simulink model "model_base_bros"  (R2017b)
settings: Solver=FixedStepDiscrete  StartTime=0.0  StopTime=inf  FixedStep=sampleTime  RelTol=1e-3
PostLoadFcn:
  | % load model parameters
  | % pname = fileparts(get_param('model_base_bros','filename'));
  | % run([pname  '\parameters_base_model_bros.m']);
  | parameters_base_model_bros;
  | 
  | % set requested state
  | set_param('model_base_bros/Requested state','Value',num2str(0));
InitFcn:
  | % load model parameters
  | % pname = fileparts(get_param('model_base_bros','filename'));
  | % run([pname  '\parameters_base_model_bros.m']);
  | parameters_base_model_bros;
  | 
  | % set requested state
  | set_param('model_base_bros/Requested state','Value',num2str(0));
StartFcn:
  | % load model parameters
  | % pname = fileparts(get_param('model_base_bros','filename'));
  | % run([pname  '\parameters_base_model_bros.m']);
  | parameters_base_model_bros;
  | 
  | % set requested state
  | set_param('model_base_bros/Requested state','Value',num2str(0));
StopFcn:
  | % switch off data logger (to hopefully avoid corrupt files). TwinCAT doesn't properly switch off the logger when shutting down the model
  | % no idea if this'll work.
  | set_param('model_base_bros/Record data (1 = yes, 0 = no)','Value',num2str(0));
values from neighbouring files (symbols this model uses):
  FFMatrix = -[0 -15; 15 0]    [parameters_base_model_bros.m]
  Lb = 0.07    [parameters_base_model_bros.m]
  Lf = 0.238    [parameters_base_model_bros.m]
  Lu = 0.153    [parameters_base_model_bros.m]
  sampleTime = 0.001    [parameters_base_model_bros.m]
undefined symbols (not defined in the file or in its folder): BROS1, BROS2
libraries: simulink x27, LibraryFM x14, VariousBlocksLibrary x7, simulink_extras x1
(part 1 of 3)
settings Model: SimulationMode=external  Creator=niekbeckers  LastModifiedBy=TCUser
settings DataIOCC: LimitDataPoints=on  SaveFormat=Array
settings OptimizationCC: BlockReduction=off  BooleanDataType=off  LocalBlockOutputs=off  LifeSpan=inf
settings DebuggingCC: SaveWithParameterizedLinksMsg=none  UnderspecifiedInitializationDetection=Classic  MergeDetectMultiDrivingBlocksExec=none  SignalResolutionControl=TryResolveAllWithWarning  SFUnexpectedBacktrackingDiag=warning  SFNoUnconditionalDefaultTransitionDiag=warning  SFExecutionAtInitializationDiag=none
settings HardwareCC: ProdBitPerPointer=32  ProdBitPerSizeT=32  ProdBitPerPtrDiffT=32  ProdLargestAtomicFloat=None  ProdIntDivRoundTo=Undefined  ProdEndianess=Unspecified  ProdWordSize=32  ProdHWDeviceType=32-bit Generic  TargetBitPerPointer=64  TargetBitPerSizeT=64  TargetBitPerPtrDiffT=64  TargetLongLongMode=on  TargetIntDivRoundTo=Zero  TargetEndianess=LittleEndian  TargetWordSize=64  TargetHWDeviceType=MATLAB Host  ProdEqTarget=off
settings ModelReferenceCC: PropagateSignalLabelsOutOfModel=off
settings RTWCC: SystemTargetFile=TwinCAT.tlc  GenCodeOnly=on  MakeCommand=make_tct  TemplateMakefile=tct_msbuild.tmf  Description=TwinCAT Target  GenerateReport=on  TargetLang=C++
settings CodeAppCC: StateflowObjectComments=on
settings STFCustomTargetCC: CompOptLevelCompliant=on  GeneratePreprocessorConditionals=Disable all  MATLABClassNameForMDSCustomization=Simulink.SoftwareTarget.TargetSpecificTriggerConfigurationBase  SystemTargetFile=TwinCAT.tlc
settings ConfigComp: CovMetricSettings=dw  CovHtmlReporting=on  CovSaveCumulativeToWorkspaceVar=on  CovSaveSingleToWorkspaceVar=on  CovExternalEMLEnable=off  CovSFcnEnable=off
settings SimscapeCC: SimscapeNormalizeSystem=off

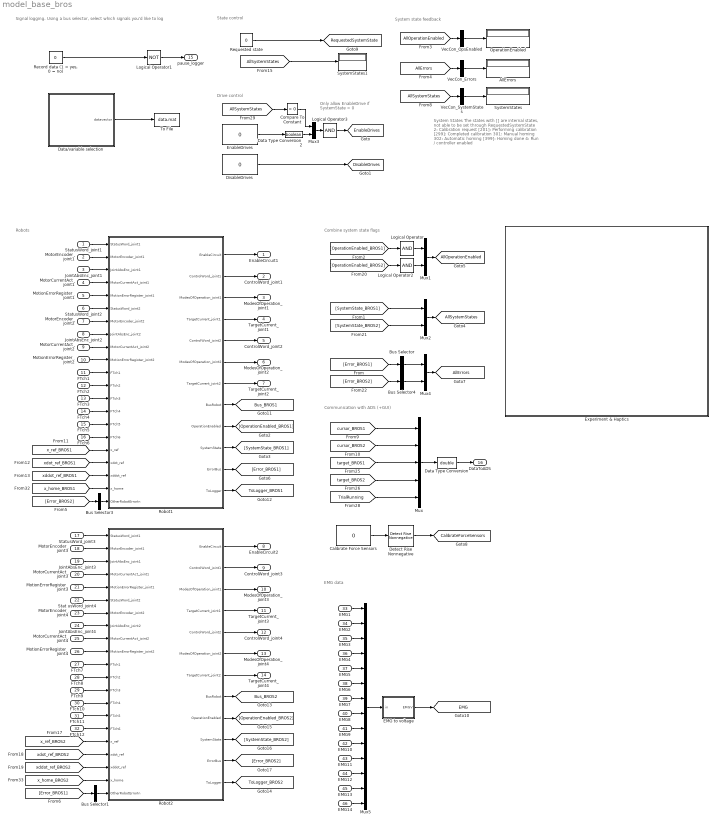
== system model_base_bros ==
  note: EMG data
  note: Drive control
  note: System state feedback
  note: Only allow EnableDrive
      | if SystemState > 0
  note: Communication with ADS (+GUI)
  note: Signal logging.
      | Using a bus selector, select which signals you'd like to log
  note: System States
      | The states with [] are internal states, not able to be set through RequestedSystemState
      | 2: Calibration request
      | [201]: Performing calibration
      | [299]: Completed calibration
      | 301: Manual homing
      | 302: Automatic homing
      | [399]: Homing done
      | 4: Run / controller enabled
  note: State control
  note: Combine system state flags
  note: Robots
  StatusWord_joint1 : Inport  OutDataTypeStr=uint16  PortDimensions=1
  MotorEncoder_joint1 : Inport  Port=2  OutDataTypeStr=int32  PortDimensions=1
  JointAbsEnc_joint1 : Inport  Port=3  OutDataTypeStr=int32  PortDimensions=1
  MotorCurrentAct_joint1 : Inport  Port=4  OutDataTypeStr=int16  PortDimensions=1
  MotionErrorRegister_joint1 : Inport  Port=5  OutDataTypeStr=uint16  PortDimensions=1
  StatusWord_joint2 : Inport  Port=6  OutDataTypeStr=uint16  PortDimensions=1
  MotorEncoder_joint2 : Inport  Port=7  OutDataTypeStr=int32  PortDimensions=1
  JointAbsEnc_joint2 : Inport  Port=8  OutDataTypeStr=int32  PortDimensions=1
  MotorCurrentAct_joint2 : Inport  Port=9  OutDataTypeStr=int16  PortDimensions=1
  MotionErrorRegister_joint2 : Inport  Port=10  OutDataTypeStr=uint16  PortDimensions=1
  FTch1 : Inport  Port=11  OutDataTypeStr=single  PortDimensions=1
  FTch2 : Inport  Port=12  OutDataTypeStr=single  PortDimensions=1
  FTch3 : Inport  Port=13  OutDataTypeStr=single  PortDimensions=1
  FTch4 : Inport  Port=14  OutDataTypeStr=single  PortDimensions=1
  FTch5 : Inport  Port=15  OutDataTypeStr=single  PortDimensions=1
  FTch6 : Inport  Port=16  OutDataTypeStr=single  PortDimensions=1
  StatusWord_joint3 : Inport  Port=17  OutDataTypeStr=uint16  PortDimensions=1
  MotorEncoder_joint3 : Inport  Port=18  OutDataTypeStr=int32  PortDimensions=1
  JointAbsEnc_joint3 : Inport  Port=19  OutDataTypeStr=int32  PortDimensions=1
  MotorCurrentAct_joint3 : Inport  Port=20  OutDataTypeStr=int16  PortDimensions=1
  MotionErrorRegister_joint3 : Inport  Port=21  OutDataTypeStr=uint16  PortDimensions=1
  Stat usWord_joint4 : Inport  Port=22  OutDataTypeStr=uint16  PortDimensions=1
  MotorEncoder_joint4 : Inport  Port=23  OutDataTypeStr=int32  PortDimensions=1
  JointAbsEnc_joint4 : Inport  Port=24  OutDataTypeStr=int32  PortDimensions=1
  MotorCurrentAct_joint4 : Inport  Port=25  OutDataTypeStr=int16  PortDimensions=1
  MotionErrorRegister_joint4 : Inport  Port=26  OutDataTypeStr=uint16  PortDimensions=1
  FTch7 : Inport  Port=27  OutDataTypeStr=single  PortDimensions=1
  FTch8 : Inport  Port=28  OutDataTypeStr=single  PortDimensions=1
  FTch9 : Inport  Port=29  OutDataTypeStr=single  PortDimensions=1
  FTch10 : Inport  Port=30  OutDataTypeStr=single  PortDimensions=1
  FTch11 : Inport  Port=31  OutDataTypeStr=single  PortDimensions=1
  FTch12 : Inport  Port=32  OutDataTypeStr=single  PortDimensions=1
  EMG1 : Inport  Port=33  OutDataTypeStr=int16  PortDimensions=1
  EMG2 : Inport  Port=34  OutDataTypeStr=int16  PortDimensions=1
  EMG3 : Inport  Port=35  OutDataTypeStr=int16  PortDimensions=1
  EMG4 : Inport  Port=36  OutDataTypeStr=int16  PortDimensions=1
  EMG5 : Inport  Port=37  OutDataTypeStr=int16  PortDimensions=1
  EMG6 : Inport  Port=38  OutDataTypeStr=int16  PortDimensions=1
  EMG7 : Inport  Port=39  OutDataTypeStr=int16  PortDimensions=1
  EMG8 : Inport  Port=40  OutDataTypeStr=int16  PortDimensions=1
  EMG9 : Inport  Port=41  OutDataTypeStr=int16  PortDimensions=1
  EMG10 : Inport  Port=42  OutDataTypeStr=int16  PortDimensions=1
  EMG11 : Inport  Port=43  OutDataTypeStr=int16  PortDimensions=1
  EMG12 : Inport  Port=44  OutDataTypeStr=int16  PortDimensions=1
  EMG13 : Inport  Port=45  OutDataTypeStr=int16  PortDimensions=1
  EMG14 : Inport  Port=46  OutDataTypeStr=int16  PortDimensions=1
  AllErrors : Display
      settings: OpenFcn=msgbox(DecodeBROSError(gcb));  Format=hex (Stored Integer)
  Bus Selector : BusSelector  OutputSignals=ErrorCodeLatched  OutputAsBus=on
  Bus Selector1 : BusSelector  OutputSignals=ErrorCode  OutputAsBus=on
  Bus Selector3 : BusSelector  OutputSignals=ErrorCode  OutputAsBus=on
  Bus Selector4 : BusSelector  OutputSignals=ErrorCodeLatched  OutputAsBus=on
  Calibrate Force Sensors : Constant  Value=0
      settings: OpenFcn=set_param(gcb,'Value','1');tname = ['toggletimer_' gcb];delete(timerfind('name',tname));t = timer('timerfcn', ['set_param(''',gcb,''',''Value'',''0'')'],'executionmode','singleshot','startdelay',1,'name',tname);start(t);
      mask Display: fprintf('PushToTrigger\n%s',get_param(gcb,'value'))
  Compare To Constant : simulink/Logic and Bit Operations/Compare To Constant  relop=>  const=0  OutDataTypeStr=boolean
  Data Type Conversion : DataTypeConversion  OutDataTypeStr=double
  Data Type Conversion2 : DataTypeConversion  OutDataTypeStr=boolean
  Data/variable selection : Subsystem
  Detect Rise Nonnegative : simulink/Logic and Bit Operations/Detect Rise Nonnegative  vinit=0  OutDataTypeStr=boolean
      settings: SourceProductName=Simulink  SourceProductBaseCode=SL
  DisableDrives : Constant  Value=0
      settings: OpenFcn=set_param(gcb,'Value','1');tname = ['toggletimer_' gcb];delete(timerfind('name',tname));t = timer('timerfcn', ['set_param(''',gcb,''',''Value'',''0'')'],'executionmode','singleshot','startdelay',1,'name',tname);start(t);
      mask Display: fprintf('PushToTrigger\n%s',get_param(gcb,'value'))
  EMG to voltage : MATLAB Function  TreatAsAtomicUnit=on
  EnableDrives : Constant  Value=0
      settings: OpenFcn=set_param(gcb,'Value','1');tname = ['toggletimer_' gcb];delete(timerfind('name',tname));t = timer('timerfcn', ['set_param(''',gcb,''',''Value'',''0'')'],'executionmode','singleshot','startdelay',1,'name',tname);start(t);
      mask Display: fprintf('PushToTrigger\n%s',get_param(gcb,'value'))
  Experiment & Haptics : Subsystem
  Logical Operator : Logic  Inputs=1  AllPortsSameDT=off  OutDataTypeStr=boolean
  Logical Operator1 : Logic  Operator=NOT  Inputs=1  AllPortsSameDT=off  OutDataTypeStr=boolean
  Logical Operator2 : Logic  Inputs=1  AllPortsSameDT=off  OutDataTypeStr=boolean
  Logical Operator3 : Logic  Inputs=1  AllPortsSameDT=off  OutDataTypeStr=boolean
  Mux : Mux  Inputs=5
  Mux{1..4} (4 alike) : Mux  Inputs=2
  Mux5 : Mux  Inputs=14
  OperationEnabled : Display
  "Record data (1 = yes, 0 = no)" : Constant  Value=0  OutDataTypeStr=boolean
  Requested state : Constant  Value=0
  Robot1 : Subsystem  mask{RobotStruct=BROS1}
      mask prompts: RobotStruct "Robot struct (data)"
  Robot2 : Subsystem  mask{RobotStruct=BROS2}
      mask prompts: RobotStruct "Robot struct (data)"
  SystemStates : Display
  SystemStates1 : Display
  To File : ToFile  Filename=data.mat  MatrixName=data
  VecCon_Errors : Concatenate  NumInputs=1
  VecCon_OpsEnabled : Concatenate  NumInputs=1
  VecCon_SystemStates : Concatenate  NumInputs=1
  EnableCircuit1 : Outport  OutDataTypeStr=boolean  PortDimensions=1
  ControlWord_joint1 : Outport  Port=2  OutDataTypeStr=uint16  PortDimensions=1
  ModesOfOperation_joint1 : Outport  Port=3  OutDataTypeStr=int8  PortDimensions=1
  TargetCurrent_joint1 : Outport  Port=4  OutDataTypeStr=int16  PortDimensions=1
  ControlWord_joint2 : Outport  Port=5  OutDataTypeStr=uint16  PortDimensions=1
  ModesOfOperation_joint2 : Outport  Port=6  OutDataTypeStr=int8  PortDimensions=1
  TargetCurrent_joint2 : Outport  Port=7  OutDataTypeStr=int16  PortDimensions=1
  EnableCircuit2 : Outport  Port=8  OutDataTypeStr=boolean  PortDimensions=1
  ControlWord_joint3 : Outport  Port=9  OutDataTypeStr=uint16  PortDimensions=1
  ModesOfOperation_joint3 : Outport  Port=10  OutDataTypeStr=int8  PortDimensions=1
  TargetCurrent_joint3 : Outport  Port=11  OutDataTypeStr=int16  PortDimensions=1
  ControlWord_joint4 : Outport  Port=12  OutDataTypeStr=uint16  PortDimensions=1
  ModesOfOperation_joint4 : Outport  Port=13  OutDataTypeStr=int8  PortDimensions=1
  TargetCurrent_joint4 : Outport  Port=14  OutDataTypeStr=int16  PortDimensions=1
  pause_logger : Outport  Port=15  OutDataTypeStr=boolean  PortDimensions=1
  DataToADS : Outport  Port=16  OutDataTypeStr=double
  tag scope: AllErrors=global, AllOperationEnabled=global, AllSystemStates=global, Bus_BROS1=global, Bus_BROS2=global, CalibrateForceSensors=global, DisableDrives=global, EMG=global, EnableDrives=global, RequestedSystemState=global, ToLogger_BROS1=global, ToLogger_BROS2=global
  wires:
  DisableDrives/1 -> [DisableDrives]
  Robot1/9(OperationEnabled) -> [OperationEnabled_BROS1]
  [AllOperationEnabled] -> VecCon_OpsEnabled/1
  Robot1/10(SystemState) -> [SystemState_BROS1]
  [SystemState_BROS1] -> Mux2/1
  Mux2/1 -> [AllSystemStates]
  Mux1/1 -> [AllOperationEnabled]
  [OperationEnabled_BROS1] -> Logical Operator/1
  Robot1/11(ErrorBus) -> [Error_BROS1]
  [Error_BROS1] -> Bus Selector/1
  [AllErrors] -> VecCon_Errors/1
  [x_ref_BROS1] -> Robot1/17(x_ref)
  [xdot_ref_BROS1] -> Robot1/18(xdot_ref)
  [xddot_ref_BROS1] -> Robot1/19(xddot_ref)
  Requested state/1 -> [RequestedSystemState]
  Robot1/8(BusRobot) -> [Bus_BROS1]
  StatusWord_joint1/1 -> Robot1/1(StatusWord_joint1)
  MotorEncoder_joint1/1 -> Robot1/2(MotorEncoder_joint1)
  JointAbsEnc_joint1/1 -> Robot1/3(JointAbsEnc_joint1)
  MotorCurrentAct_joint1/1 -> Robot1/4(MotorCurrentAct_joint1)
  StatusWord_joint2/1 -> Robot1/6(StatusWord_joint2)
  MotorEncoder_joint2/1 -> Robot1/7(MotorEncoder_joint2)
  JointAbsEnc_joint2/1 -> Robot1/8(JointAbsEnc_joint2)
  MotorCurrentAct_joint2/1 -> Robot1/9(MotorCurrentAct_joint2)
  FTch1/1 -> Robot1/11(FTch1)
  FTch2/1 -> Robot1/12(FTch2)
  FTch3/1 -> Robot1/13(FTch3)
  FTch4/1 -> Robot1/14(FTch4)
  FTch5/1 -> Robot1/15(FTch5)
  FTch6/1 -> Robot1/16(FTch6)
  Robot1/2(ControlWord_joint1) -> ControlWord_joint1/1
  Robot1/3(ModesOfOperation_joint1) -> ModesOfOperation_joint1/1
  Robot1/4(TargetCurrent_joint1) -> TargetCurrent_joint1/1
  Robot1/7(TargetCurrent_joint2) -> TargetCurrent_joint2/1
  Robot1/6(ModesOfOperation_joint2) -> ModesOfOperation_joint2/1
  Robot1/5(ControlWord_joint2) -> ControlWord_joint2/1
  Robot1/12(ToLogger) -> [ToLogger_BROS1]
  Logical Operator/1 -> Mux1/1
  [AllSystemStates] -> SystemStates1/1
  Logical Operator1/1 -> pause_logger/1
  Robot2/9(OperationEnabled) -> [OperationEnabled_BROS2]
  Robot2/10(SystemState) -> [SystemState_BROS2]
  Robot2/11(ErrorBus) -> [Error_BROS2]
  [x_ref_BROS2] -> Robot2/17(x_ref)
  [xdot_ref_BROS2] -> Robot2/18(xdot_ref)
  [xddot_ref_BROS2] -> Robot2/19(xddot_ref)
  Robot2/8(BusRobot) -> [Bus_BROS2]
  StatusWord_joint3/1 -> Robot2/1(StatusWord_joint1)
  MotorEncoder_joint3/1 -> Robot2/2(MotorEncoder_joint1)
  JointAbsEnc_joint3/1 -> Robot2/3(JointAbsEnc_joint1)
  MotorCurrentAct_joint3/1 -> Robot2/4(MotorCurrentAct_joint1)
  Stat usWord_joint4/1 -> Robot2/6(StatusWord_joint2)
  MotorEncoder_joint4/1 -> Robot2/7(MotorEncoder_joint2)
  MotorCurrentAct_joint4/1 -> Robot2/9(MotorCurrentAct_joint2)
  FTch7/1 -> Robot2/11(FTch1)
  FTch8/1 -> Robot2/12(FTch2)
  FTch9/1 -> Robot2/13(FTch3)
  FTch10/1 -> Robot2/14(FTch4)
  FTch12/1 -> Robot2/16(FTch6)
  Robot2/1(EnableCircuit) -> EnableCircuit2/1
  Robot2/2(ControlWord_joint1) -> ControlWord_joint3/1
  Robot2/3(ModesOfOperation_joint1) -> ModesOfOperation_joint3/1
  Robot2/7(TargetCurrent_joint2) -> TargetCurrent_joint4/1
  Robot2/6(ModesOfOperation_joint2) -> ModesOfOperation_joint4/1
  Robot2/5(ControlWord_joint2) -> ControlWord_joint4/1
  Robot2/12(ToLogger) -> [ToLogger_BROS2]
  [OperationEnabled_BROS2] -> Logical Operator2/1
  Logical Operator2/1 -> Mux1/2
  [SystemState_BROS2] -> Mux2/2
  Mux4/1 -> [AllErrors]
  Bus Selector/1 -> Mux4/1
  [Error_BROS2] -> Bus Selector4/1
  Bus Selector4/1 -> Mux4/2
  Robot1/1(EnableCircuit) -> EnableCircuit1/1
  Robot2/4(TargetCurrent_joint1) -> TargetCurrent_joint3/1
  JointAbsEnc_joint4/1 -> Robot2/8(JointAbsEnc_joint2)
  FTch11/1 -> Robot2/15(FTch5)
  [Error_BROS2] -> Bus Selector3/1
  [Error_BROS1] -> Bus Selector1/1
  Bus Selector1/1 -> Robot2/21(OtherRobotErrorIn)
  Bus Selector3/1 -> Robot1/21(OtherRobotErrorIn)
  VecCon_Errors/1 -> AllErrors/1
  [AllSystemStates] -> VecCon_SystemStates/1
  VecCon_SystemStates/1 -> SystemStates/1
  VecCon_OpsEnabled/1 -> OperationEnabled/1
  Mux/1 -> Data Type Conversion/1
  Data Type Conversion/1 -> DataToADS/1
  [cursor_BROS1] -> Mux/1
  [cursor_BROS2] -> Mux/2
  [target_BROS1] -> Mux/3
  [target_BROS2] -> Mux/4
  [TrialRunning] -> Mux/5
  Calibrate Force Sensors/1 -> Detect Rise Nonnegative/1
  Detect Rise Nonnegative/1 -> [CalibrateForceSensors]
  [AllSystemStates] -> Compare To Constant/1
  Logical Operator3/1 -> [EnableDrives]
  EnableDrives/1 -> Data Type Conversion2/1
  Compare To Constant/1 -> Mux3/1
  Mux3/1 -> Logical Operator3/1
  Data Type Conversion2/1 -> Mux3/2
  [x_home_BROS1] -> Robot1/20(x_home)
  [x_home_BROS2] -> Robot2/20(x_home)
  Data/variable selection/1(datavector) -> To File/1
  MotionErrorRegister_joint1/1 -> Robot1/5(MotionErrorRegister_joint1)
  MotionErrorRegister_joint2/1 -> Robot1/10(MotionErrorRegister_joint2)
  MotionErrorRegister_joint3/1 -> Robot2/5(MotionErrorRegister_joint1)
  MotionErrorRegister_joint4/1 -> Robot2/10(MotionErrorRegister_joint2)
  EMG1/1 -> Mux5/1
  EMG2/1 -> Mux5/2
  EMG3/1 -> Mux5/3
  EMG4/1 -> Mux5/4
  EMG5/1 -> Mux5/5
  EMG6/1 -> Mux5/6
  EMG7/1 -> Mux5/7
  EMG8/1 -> Mux5/8
  EMG9/1 -> Mux5/9
  EMG10/1 -> Mux5/10
  EMG11/1 -> Mux5/11
  EMG12/1 -> Mux5/12
  Mux5/1 -> EMG to voltage/1(in)
  EMG to voltage/1(EMGV) -> [EMG]
  EMG13/1 -> Mux5/13
  EMG14/1 -> Mux5/14
  "Record data (1 = yes, 0 = no)"/1 -> Logical Operator1/1

== system model_base_bros/Data//variable selection ==
  Bus to Vector : BusToVector
  Bus to Vector3 : BusToVector
  BusSelectorLoggerBROS1 : BusSelector  OutputSignals=SystemState,qJointSpace.q_AbsEnc,qJointSpace.qdot_AbsEnc,qJointSpace.q_IncEnc,qJointSpace.qdot_IncEnc,xOpSpace.x_AbsEnc,xOpSpace.xdot_AbsEnc,xOpSpace.x,xOpSpace.xdot,Controller_ToLogger.x_ref,Controller_ToLogger.xdot_ref,Controller_ToLogger.xddot_ref,qJointSpace.JointTorque_Nm,BusFTSensor.ForcesOpSpace  OutputAsBus=on
  BusSelectorLoggerBROS2 : BusSelector  OutputSignals=SystemState,qJointSpace.q_AbsEnc,qJointSpace.qdot_AbsEnc,qJointSpace.q_IncEnc,qJointSpace.qdot_IncEnc,xOpSpace.x_AbsEnc,xOpSpace.xdot_AbsEnc,xOpSpace.x,xOpSpace.xdot,Controller_ToLogger.x_ref,Controller_ToLogger.xdot_ref,Controller_ToLogger.xddot_ref,qJointSpace.JointTorque_Nm,BusFTSensor.ForcesOpSpace  OutputAsBus=on
  Constant : Constant  Value=0
  Mux : Mux  Inputs=6
  Mux5 : Mux  Inputs=13
  datavector : Outport
  wires:
  BusSelectorLoggerBROS1/1 -> Bus to Vector/1
  [ToLogger_BROS1] -> BusSelectorLoggerBROS1/1
  Bus to Vector3/1 -> Mux5/2
  BusSelectorLoggerBROS2/1 -> Bus to Vector3/1
  Bus to Vector/1 -> Mux5/1
  [ToLogger_BROS2] -> BusSelectorLoggerBROS2/1
  Mux5/1 -> datavector/1
  [AllErrors] -> Mux5/7
  [cursor_BROS2] -> Mux5/6
  [target_BROS1] -> Mux5/3
  [AdmittanceData] -> Mux5/9
  [target_BROS2] -> Mux5/4
  [ExpData] -> Mux5/8
  [cursor_BROS1] -> Mux5/5
  [target_vel_BROS1] -> Mux5/10
  [target_vel_BROS2] -> Mux5/11
  Constant/1 -> Mux/6, Mux/5, Mux/4, Mux/3, Mux/2, Mux/1
  Mux/1 -> Mux5/12
  [EMG] -> Mux5/13

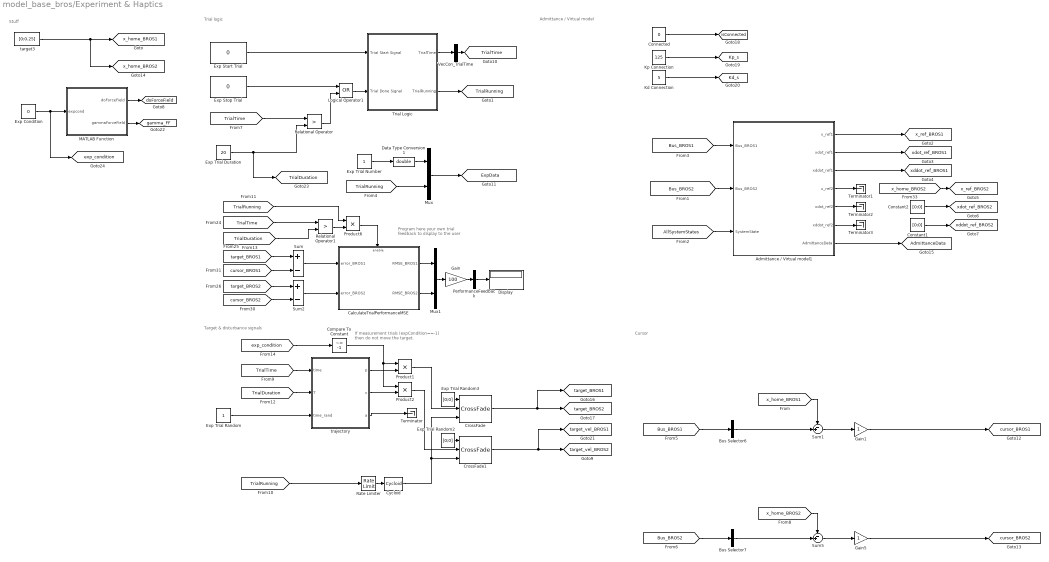
== system model_base_bros/Experiment & Haptics ==
  note: If measurement trials (expCondition==-1)
      | then do not move the target.
  note: Stuff
  note: Cursor
  note: Program here your own trial
      | feedback to display to the user
  note: Target & disturbance signals
  note: Trial logic
  note: Admittance / Virtual model
  Admittance / Virtual model1 : Subsystem
  Bus Selector6 : BusSelector  OutputSignals=xOpSpace.x  OutputAsBus=on
  Bus Selector7 : BusSelector  OutputSignals=xOpSpace.x  OutputAsBus=on
  CalculateTrialPerformanceMSE : Subsystem
  Compare To Constant : simulink/Logic and Bit Operations/Compare To Constant  relop=~=  const=-1  OutDataTypeStr=boolean
  Connected : Constant  Value=0  OutDataTypeStr=boolean
  Constant1 : Constant  Value=[0;0]
  Constant2 : Constant  Value=[0;0]
  CrossFade : VariousBlocksLibrary/Various/CrossFade
  CrossFade1 : VariousBlocksLibrary/Various/CrossFade
  Cycloid : VariousBlocksLibrary/Various/Cycloid
  Data Type Conversion1 : DataTypeConversion  OutDataTypeStr=double
  Display : Display
  Exp Condition : Constant  Value=0  OutDataTypeStr=int32
  Exp Start Trial : Constant  Value=0
      settings: OpenFcn=set_param(gcb,'Value','1');tname = ['toggletimer_' gcb];delete(timerfind('name',tname));t = timer('timerfcn', ['set_param(''',gcb,''',''Value'',''0'')'],'executionmode','singleshot','startdelay',1,'name',tname);start(t);
      mask Display: fprintf('PushToTrigger\n%s',get_param(gcb,'value'))
  Exp Stop Trial : Constant  Value=0
      settings: OpenFcn=set_param(gcb,'Value','1');tname = ['toggletimer_' gcb];delete(timerfind('name',tname));t = timer('timerfcn', ['set_param(''',gcb,''',''Value'',''0'')'],'executionmode','singleshot','startdelay',1,'name',tname);start(t);
      mask Display: fprintf('PushToTrigger\n%s',get_param(gcb,'value'))
  Exp Trial Duration : Constant  Value=20  OutDataTypeStr=double
  Exp Trial Number : Constant  OutDataTypeStr=int32
  Exp Trial Random : Constant  OutDataTypeStr=double
  Exp Trial Random2 : Constant  Value=[0;0]  OutDataTypeStr=int32
  Exp Trial Random3 : Constant  Value=[0;0]  OutDataTypeStr=int32
  Gain : Gain  Gain=100
  Gain1 : Gain
  Gain5 : Gain
  Kd Connection : Constant  Value=5  OutDataTypeStr=double
  Kp Connection : Constant  Value=125  OutDataTypeStr=double
  Logical Operator1 : Logic  Operator=OR  AllPortsSameDT=off  OutDataTypeStr=boolean
  MATLAB Function : MATLAB Function  TreatAsAtomicUnit=on
  Mux : Mux  Inputs=2
  Mux1 : Mux  Inputs=2
  PerformanceFeedback : Concatenate  NumInputs=1
  Product1 : Product
  Product2 : Product
  Product6 : Product
  Rate Limiter : RateLimiter  RisingSlewLimit=1/2.0  FallingSlewLimit=-1/2.0  SampleTimeMode=inherited
  Relational Operator : RelationalOperator  Operator=>  OutDataTypeStr=boolean  RndMeth=Simplest
  Relational Operator1 : RelationalOperator  Operator=>  OutDataTypeStr=boolean  RndMeth=Simplest
  Sum : Sum  Inputs=+-
  Sum1 : Sum  Inputs=-+|
  Sum2 : Sum  Inputs=+-
  Sum5 : Sum  Inputs=-+|
  Terminator{,1..3} (4 alike) : Terminator
  Trial Logic : Subsystem
  VecCon_TrialTime : Concatenate  NumInputs=1
  target3 : Constant  Value=[0;0.25]
  trajectory : MATLAB Function  TreatAsAtomicUnit=on
  tag scope: AdmittanceData=global, ExpData=global, Kd_s=global, Kp_s=global, TrialDuration=global, TrialRunning=global, TrialTime=global, cursor_BROS1=global, cursor_BROS2=global, doForceField=global, exp_condition=global, gamma_FF=global, isConnected=global, target_BROS1=global, target_BROS2=global, target_vel_BROS1=global, target_vel_BROS2=global, x_home_BROS1=global, x_home_BROS2=global, x_ref_BROS1=global, x_ref_BROS2=global, xddot_ref_BROS1=global, xddot_ref_BROS2=global, xdot_ref_BROS1=global, xdot_ref_BROS2=global
  wires:
  Kp Connection/1 -> [Kp_s]
  Mux/1 -> [ExpData]
  Exp Trial Number/1 -> Data Type Conversion1/1
  [TrialRunning] -> Mux/2
  Connected/1 -> [isConnected]
  [TrialTime] -> trajectory/1(time)
  Data Type Conversion1/1 -> Mux/1
  Kd Connection/1 -> [Kd_s]
  [Bus_BROS1] -> Admittance / Virtual model1/1(Bus_BROS1)
  target3/1 -> [x_home_BROS2], [x_home_BROS1]
  Exp Start Trial/1 -> Trial Logic/1(Trial Start Signal)
  Trial Logic/1(TrialTime) -> VecCon_TrialTime/1
  Trial Logic/2(TrialRunning) -> [TrialRunning]
  [Bus_BROS2] -> Admittance / Virtual model1/2(Bus_BROS2)
  PerformanceFeedback/1 -> Display/1
  Admittance / Virtual model1/7(AdmittanceData) -> [AdmittanceData]
  [AllSystemStates] -> Admittance / Virtual model1/3(SystemState)
  Mux1/1 -> Gain/1
  [target_BROS1] -> Sum/1
  [cursor_BROS1] -> Sum/2
  [target_BROS2] -> Sum2/1
  [cursor_BROS2] -> Sum2/2
  Sum/1 -> CalculateTrialPerformanceMSE/1(error_BROS1)
  Sum2/1 -> CalculateTrialPerformanceMSE/2(error_BROS2)
  CalculateTrialPerformanceMSE/1(RMSE_BROS1) -> Mux1/1
  CalculateTrialPerformanceMSE/2(RMSE_BROS2) -> Mux1/2
  Gain/1 -> PerformanceFeedback/1
  Rate Limiter/1 -> Cycloid/1
  [TrialRunning] -> Rate Limiter/1
  Exp Trial Random3/1 -> CrossFade/1
  Exp Trial Duration/1 -> [TrialDuration], Relational Operator/2
  [TrialTime] -> Relational Operator/1
  CrossFade/1 -> [target_BROS2], [target_BROS1]
  [TrialDuration] -> trajectory/2(T)
  CrossFade1/1 -> [target_vel_BROS1], [target_vel_BROS2]
  Exp Trial Random2/1 -> CrossFade1/1
  Exp Condition/1 -> [exp_condition], MATLAB Function/1(expcond)
  [Bus_BROS1] -> Bus Selector6/1
  [Bus_BROS2] -> Bus Selector7/1
  trajectory/3(a) -> Terminator/1
  Admittance / Virtual model1/1(x_ref1) -> [x_ref_BROS1]
  Admittance / Virtual model1/2(xdot_ref1) -> [xdot_ref_BROS1]
  Admittance / Virtual model1/3(xddot_ref1) -> [xddot_ref_BROS1]
  Exp Trial Random/1 -> trajectory/3(time_rand)
  Cycloid/1 -> CrossFade1/3, CrossFade/3
  [x_home_BROS1] -> Sum1/1
  [x_home_BROS2] -> Sum5/1
  Bus Selector7/1 -> Sum5/2
  Gain1/1 -> [cursor_BROS1]
  Bus Selector6/1 -> Sum1/2
  Sum1/1 -> Gain1/1
  Sum5/1 -> Gain5/1
  Gain5/1 -> [cursor_BROS2]
  VecCon_TrialTime/1 -> [TrialTime]
  Logical Operator1/1 -> Trial Logic/2(Trial Done Signal)
  Relational Operator/1 -> Logical Operator1/2
  Exp Stop Trial/1 -> Logical Operator1/1
  [TrialDuration] -> Relational Operator1/2
  [TrialTime] -> Relational Operator1/1
  Relational Operator1/1 -> Product6/2
  [TrialRunning] -> Product6/1
  Product6/1 -> CalculateTrialPerformanceMSE/Enable
  Constant2/1 -> [xdot_ref_BROS2]
  Constant1/1 -> [xddot_ref_BROS2]
  [x_home_BROS2] -> [x_ref_BROS2]
  Admittance / Virtual model1/4(x_ref2) -> Terminator1/1
  Admittance / Virtual model1/6(xddot_ref2) -> Terminator3/1
  Admittance / Virtual model1/5(xdot_ref2) -> Terminator2/1
  MATLAB Function/2(gammaForceField) -> [gamma_FF]
  MATLAB Function/1(doForceField) -> [doForceField]
  trajectory/1(p) -> Product1/2
  Product1/1 -> CrossFade/2
  trajectory/2(v) -> Product2/2
  Product2/1 -> CrossFade1/2
  Compare To Constant/1 -> Product2/1, Product1/1
  [exp_condition] -> Compare To Constant/1

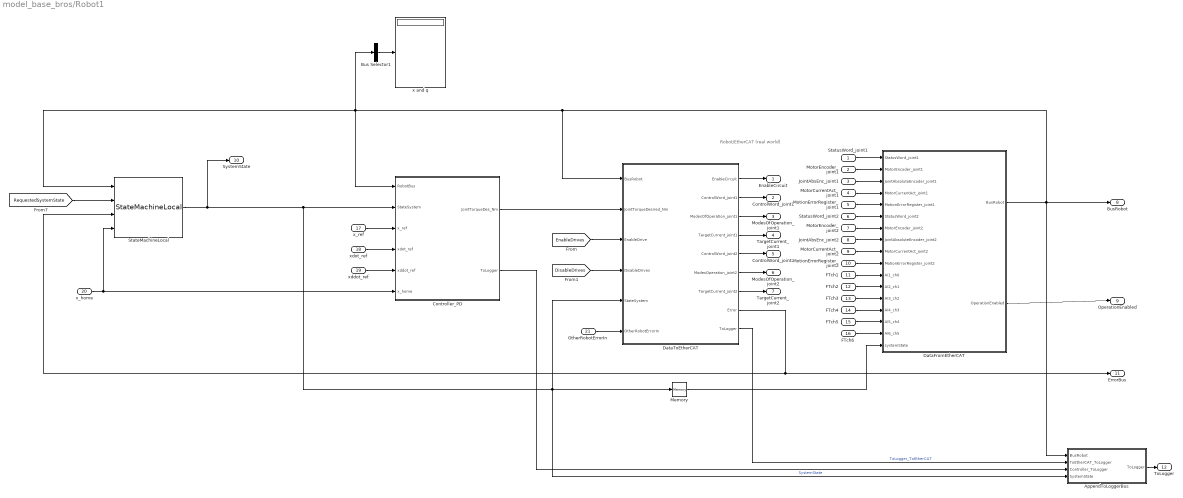
== system model_base_bros/Robot1 ==
  note: Robot/EtherCAT (real world)
  StatusWord_joint1 : Inport
  MotorEncoder_joint1 : Inport  Port=2
  JointAbsEnc_joint1 : Inport  Port=3
  MotorCurrentAct_joint1 : Inport  Port=4
  MotionErrorRegister_joint1 : Inport  Port=5  OutDataTypeStr=uint16
  StatusWord_joint2 : Inport  Port=6
  MotorEncoder_joint2 : Inport  Port=7
  JointAbsEnc_joint2 : Inport  Port=8
  MotorCurrentAct_joint2 : Inport  Port=9
  MotionErrorRegister_joint2 : Inport  Port=10  OutDataTypeStr=uint16
  FTch1 : Inport  Port=11
  FTch2 : Inport  Port=12
  FTch3 : Inport  Port=13
  FTch4 : Inport  Port=14
  FTch5 : Inport  Port=15
  FTch6 : Inport  Port=16
  x_ref : Inport  Port=17
  xdot_ref : Inport  Port=18
  xddot_ref : Inport  Port=19
  x_home : Inport  Port=20
  OtherRobotErrorIn : Inport  Port=21
  AppendToLoggerBus : Subsystem
  Bus Selector1 : BusSelector  OutputSignals=qJointSpace.q_AbsEnc,qJointSpace.qdot_AbsEnc,xOpSpace.x,BusActuators.BusActuator1.JointPosition_AbsEnc_rad,BusActuators.BusActuator2.JointPosition_AbsEnc_rad  OutputAsBus=on
  Controller_PD : Subsystem
  DataFromEtherCAT : Subsystem
  DataToEtherCAT : Subsystem
  Memory : Memory
  StateMachineLocal : LibraryFM/StateMachineLocal
  x and q : Display
  EnableCircuit : Outport
  ControlWord_joint1 : Outport  Port=2
  ModesOfOperation_joint1 : Outport  Port=3
  TargetCurrent_joint1 : Outport  Port=4
  ControlWord_joint2 : Outport  Port=5
  ModesOfOperation_joint2 : Outport  Port=6
  TargetCurrent_joint2 : Outport  Port=7
  BusRobot : Outport  Port=8
  OperationEnabled : Outport  Port=9
  SystemState : Outport  Port=10
  ErrorBus : Outport  Port=11
  ToLogger : Outport  Port=12
  wires:
  xddot_ref/1 -> Controller_PD/5(xddot_ref)
  xdot_ref/1 -> Controller_PD/4(xdot_ref)
  x_ref/1 -> Controller_PD/3(x_ref)
  DataToEtherCAT/7(TargetCurrent_joint2) -> TargetCurrent_joint2/1
  FTch2/1 -> DataFromEtherCAT/12(AI2_ch1)
  MotorCurrentAct_joint1/1 -> DataFromEtherCAT/4(MotorCurrentAct_joint1)
  MotorEncoder_joint2/1 -> DataFromEtherCAT/7(MotorEncoder_joint2)
  JointAbsEnc_joint1/1 -> DataFromEtherCAT/3(JointAbsoluteEncoder_joint1)
  DataToEtherCAT/3(ModesOfOperation_joint1) -> ModesOfOperation_joint1/1
  DataToEtherCAT/1(EnableCircuit) -> EnableCircuit/1
  FTch1/1 -> DataFromEtherCAT/11(AI1_ch0)
  StateMachineLocal/1 -> Controller_PD/2(StateSystem), DataToEtherCAT/5(StateSystem), Memory/1, AppendToLoggerBus/4(SystemState), SystemState/1  "SystemState"
  DataToEtherCAT/2(ControlWord_joint1) -> ControlWord_joint1/1
  DataToEtherCAT/8(Error) -> StateMachineLocal/3, ErrorBus/1
  DataFromEtherCAT/1(BusRobot) -> AppendToLoggerBus/1(BusRobot), Controller_PD/1(RobotBus), Bus Selector1/1, StateMachineLocal/1, DataToEtherCAT/1(BusRobot), BusRobot/1
  [RequestedSystemState] -> StateMachineLocal/2
  Controller_PD/1(JointTorqueDes_Nm) -> DataToEtherCAT/2(JointTorqueDesired_Nm)
  [DisableDrives] -> DataToEtherCAT/4(DisableDrives)
  [EnableDrives] -> DataToEtherCAT/3(EnableDrive)
  MotorCurrentAct_joint2/1 -> DataFromEtherCAT/9(MotorCurrentAct_joint2)
  DataToEtherCAT/4(TargetCurrent_joint1) -> TargetCurrent_joint1/1
  FTch5/1 -> DataFromEtherCAT/15(AI5_ch4)
  JointAbsEnc_joint2/1 -> DataFromEtherCAT/8("JointAbsoluteEncoder_joint2 ")
  MotorEncoder_joint1/1 -> DataFromEtherCAT/2(MotorEncoder_joint1)
  DataToEtherCAT/5(ControlWord_joint2) -> ControlWord_joint2/1
  DataToEtherCAT/6(ModesOperation_joint2) -> ModesOfOperation_joint2/1
  StatusWord_joint1/1 -> DataFromEtherCAT/1(StatusWord_joint1)
  StatusWord_joint2/1 -> DataFromEtherCAT/6(StatusWord_joint2)
  FTch6/1 -> DataFromEtherCAT/16(AI6_ch5)
  FTch4/1 -> DataFromEtherCAT/14(AI4_ch3)
  FTch3/1 -> DataFromEtherCAT/13(AI3_ch2)
  DataFromEtherCAT/2(OperationEnabled) -> OperationEnabled/1
  Bus Selector1/1 -> x and q/1
  Controller_PD/2(ToLogger) -> AppendToLoggerBus/3(Controller_ToLogger)
  DataToEtherCAT/9(ToLogger) -> AppendToLoggerBus/2(ToEtherCAT_ToLogger)  "ToLogger_ToEtherCAT"
  AppendToLoggerBus/1(ToLogger) -> ToLogger/1
  Memory/1 -> DataFromEtherCAT/17(systemState)
  OtherRobotErrorIn/1 -> DataToEtherCAT/6(OtherRobotErrorIn)
  x_home/1 -> StateMachineLocal/4, Controller_PD/6(x_home)
  MotionErrorRegister_joint1/1 -> DataFromEtherCAT/5(MotionErrorRegister_joint1)
  MotionErrorRegister_joint2/1 -> DataFromEtherCAT/10(MotionErrorRegister_joint2)

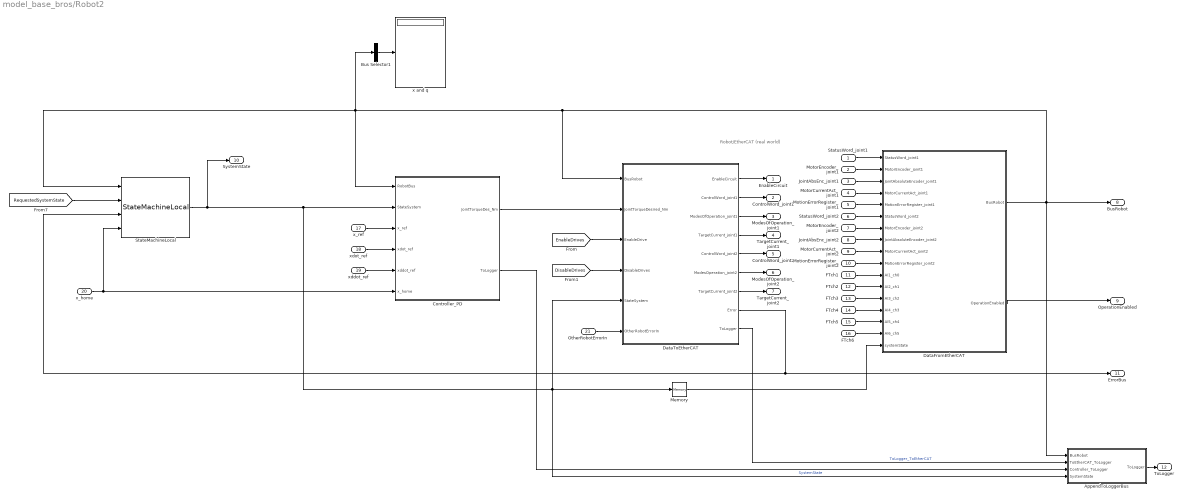
== system model_base_bros/Robot2 ==
  note: Robot/EtherCAT (real world)
  StatusWord_joint1 : Inport
  MotorEncoder_joint1 : Inport  Port=2
  JointAbsEnc_joint1 : Inport  Port=3
  MotorCurrentAct_joint1 : Inport  Port=4
  MotionErrorRegister_joint1 : Inport  Port=5  OutDataTypeStr=uint16
  StatusWord_joint2 : Inport  Port=6
  MotorEncoder_joint2 : Inport  Port=7
  JointAbsEnc_joint2 : Inport  Port=8
  MotorCurrentAct_joint2 : Inport  Port=9
  MotionErrorRegister_joint2 : Inport  Port=10  OutDataTypeStr=uint16
  FTch1 : Inport  Port=11
  FTch2 : Inport  Port=12
  FTch3 : Inport  Port=13
  FTch4 : Inport  Port=14
  FTch5 : Inport  Port=15
  FTch6 : Inport  Port=16
  x_ref : Inport  Port=17
  xdot_ref : Inport  Port=18
  xddot_ref : Inport  Port=19
  x_home : Inport  Port=20
  OtherRobotErrorIn : Inport  Port=21
  AppendToLoggerBus : Subsystem
  Bus Selector1 : BusSelector  OutputSignals=qJointSpace.q_AbsEnc,qJointSpace.qdot_AbsEnc,xOpSpace.x,BusActuators.BusActuator1.JointPosition_AbsEnc_rad,BusActuators.BusActuator2.JointPosition_AbsEnc_rad  OutputAsBus=on
  Controller_PD : Subsystem
  DataFromEtherCAT : Subsystem
  DataToEtherCAT : Subsystem
  Memory : Memory
  StateMachineLocal : LibraryFM/StateMachineLocal
  x and q : Display
  EnableCircuit : Outport
  ControlWord_joint1 : Outport  Port=2
  ModesOfOperation_joint1 : Outport  Port=3
  TargetCurrent_joint1 : Outport  Port=4
  ControlWord_joint2 : Outport  Port=5
  ModesOfOperation_joint2 : Outport  Port=6
  TargetCurrent_joint2 : Outport  Port=7
  BusRobot : Outport  Port=8
  OperationEnabled : Outport  Port=9
  SystemState : Outport  Port=10
  ErrorBus : Outport  Port=11
  ToLogger : Outport  Port=12
  wires:
  xddot_ref/1 -> Controller_PD/5(xddot_ref)
  xdot_ref/1 -> Controller_PD/4(xdot_ref)
  x_ref/1 -> Controller_PD/3(x_ref)
  DataToEtherCAT/7(TargetCurrent_joint2) -> TargetCurrent_joint2/1
  FTch2/1 -> DataFromEtherCAT/12(AI2_ch1)
  MotorCurrentAct_joint1/1 -> DataFromEtherCAT/4(MotorCurrentAct_joint1)
  MotorEncoder_joint2/1 -> DataFromEtherCAT/7(MotorEncoder_joint2)
  JointAbsEnc_joint1/1 -> DataFromEtherCAT/3(JointAbsoluteEncoder_joint1)
  DataToEtherCAT/3(ModesOfOperation_joint1) -> ModesOfOperation_joint1/1
  DataToEtherCAT/1(EnableCircuit) -> EnableCircuit/1
  FTch1/1 -> DataFromEtherCAT/11(AI1_ch0)
  StateMachineLocal/1 -> Controller_PD/2(StateSystem), DataToEtherCAT/5(StateSystem), Memory/1, AppendToLoggerBus/4(SystemState), SystemState/1  "SystemState"
  DataToEtherCAT/2(ControlWord_joint1) -> ControlWord_joint1/1
  DataToEtherCAT/8(Error) -> StateMachineLocal/3, ErrorBus/1
  DataFromEtherCAT/1(BusRobot) -> AppendToLoggerBus/1(BusRobot), Controller_PD/1(RobotBus), Bus Selector1/1, StateMachineLocal/1, DataToEtherCAT/1(BusRobot), BusRobot/1
  [RequestedSystemState] -> StateMachineLocal/2
  Controller_PD/1(JointTorqueDes_Nm) -> DataToEtherCAT/2(JointTorqueDesired_Nm)
  [DisableDrives] -> DataToEtherCAT/4(DisableDrives)
  [EnableDrives] -> DataToEtherCAT/3(EnableDrive)
  MotorCurrentAct_joint2/1 -> DataFromEtherCAT/9(MotorCurrentAct_joint2)
  DataToEtherCAT/4(TargetCurrent_joint1) -> TargetCurrent_joint1/1
  FTch5/1 -> DataFromEtherCAT/15(AI5_ch4)
  JointAbsEnc_joint2/1 -> DataFromEtherCAT/8("JointAbsoluteEncoder_joint2 ")
  MotorEncoder_joint1/1 -> DataFromEtherCAT/2(MotorEncoder_joint1)
  DataToEtherCAT/5(ControlWord_joint2) -> ControlWord_joint2/1
  DataToEtherCAT/6(ModesOperation_joint2) -> ModesOfOperation_joint2/1
  StatusWord_joint1/1 -> DataFromEtherCAT/1(StatusWord_joint1)
  StatusWord_joint2/1 -> DataFromEtherCAT/6(StatusWord_joint2)
  FTch6/1 -> DataFromEtherCAT/16(AI6_ch5)
  FTch4/1 -> DataFromEtherCAT/14(AI4_ch3)
  FTch3/1 -> DataFromEtherCAT/13(AI3_ch2)
  DataFromEtherCAT/2(OperationEnabled) -> OperationEnabled/1
  Bus Selector1/1 -> x and q/1
  Controller_PD/2(ToLogger) -> AppendToLoggerBus/3(Controller_ToLogger)
  DataToEtherCAT/9(ToLogger) -> AppendToLoggerBus/2(ToEtherCAT_ToLogger)  "ToLogger_ToEtherCAT"
  AppendToLoggerBus/1(ToLogger) -> ToLogger/1
  Memory/1 -> DataFromEtherCAT/17(systemState)
  OtherRobotErrorIn/1 -> DataToEtherCAT/6(OtherRobotErrorIn)
  x_home/1 -> StateMachineLocal/4, Controller_PD/6(x_home)
  MotionErrorRegister_joint1/1 -> DataFromEtherCAT/5(MotionErrorRegister_joint1)
  MotionErrorRegister_joint2/1 -> DataFromEtherCAT/10(MotionErrorRegister_joint2)

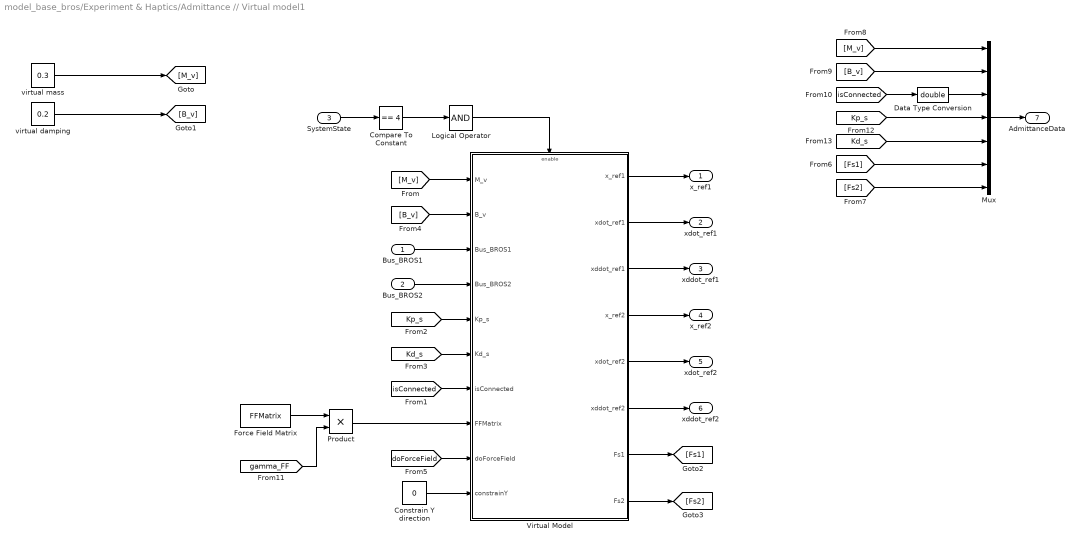
== system model_base_bros/Experiment & Haptics/Admittance // Virtual model1 ==
  Bus_BROS1 : Inport
  Bus_BROS2 : Inport  Port=2
  SystemState : Inport  Port=3
  Compare To Constant : simulink/Logic and Bit Operations/Compare To Constant  relop===  const=4  OutDataTypeStr=boolean
  Constrain Y direction : Constant  Value=0
  Data Type Conversion : DataTypeConversion  OutDataTypeStr=double
  Force Field Matrix : Constant  Value=FFMatrix  OutDataTypeStr=double
  Logical Operator : Logic  Inputs=1  AllPortsSameDT=off  OutDataTypeStr=boolean
  Mux : Mux  Inputs=7
  Product : Product
  Virtual Model : Subsystem
  virtual damping : Constant  Value=0.2
  virtual mass : Constant  Value=0.3
  x_ref1 : Outport
  xdot_ref1 : Outport  Port=2
  xddot_ref1 : Outport  Port=3
  x_ref2 : Outport  Port=4
  xdot_ref2 : Outport  Port=5
  xddot_ref2 : Outport  Port=6
  AdmittanceData : Outport  Port=7
  wires:
  virtual mass/1 -> [M_v]
  virtual damping/1 -> [B_v]
  Mux/1 -> AdmittanceData/1
  [Kd_s] -> Mux/5
  [Kp_s] -> Mux/4
  [isConnected] -> Data Type Conversion/1
  [B_v] -> Mux/2
  [M_v] -> Mux/1
  [M_v] -> Virtual Model/1(M_v)
  [B_v] -> Virtual Model/2(B_v)
  Bus_BROS1/1 -> Virtual Model/3(Bus_BROS1)
  Bus_BROS2/1 -> Virtual Model/4(Bus_BROS2)
  [Kp_s] -> Virtual Model/5(Kp_s)
  [Kd_s] -> Virtual Model/6(Kd_s)
  [isConnected] -> Virtual Model/7(isConnected)
  Virtual Model/1(x_ref1) -> x_ref1/1
  Virtual Model/2(xdot_ref1) -> xdot_ref1/1
  Virtual Model/3(xddot_ref1) -> xddot_ref1/1
  Virtual Model/4(x_ref2) -> x_ref2/1
  Virtual Model/5(xdot_ref2) -> xdot_ref2/1
  Virtual Model/6(xddot_ref2) -> xddot_ref2/1
  SystemState/1 -> Compare To Constant/1
  Compare To Constant/1 -> Logical Operator/1
  Logical Operator/1 -> Virtual Model/Enable
  Data Type Conversion/1 -> Mux/3
  [doForceField] -> Virtual Model/9(doForceField)
  [Fs1] -> Mux/6
  Virtual Model/7(Fs1) -> [Fs1]
  [Fs2] -> Mux/7
  Virtual Model/8(Fs2) -> [Fs2]
  Constrain Y direction/1 -> Virtual Model/10(constrainY)
  Force Field Matrix/1 -> Product/1
  Product/1 -> Virtual Model/8(FFMatrix)
  [gamma_FF] -> Product/2

== system model_base_bros/Experiment & Haptics/CalculateTrialPerformanceMSE ==
  note: To check: do persistents get reset in an enabled block?
  error_BROS1 : Inport
  error_BROS2 : Inport  Port=2
  Enable : EnablePort  StatesWhenEnabling=reset
  Calc_RMSE_BROS1 : MATLAB Function  TreatAsAtomicUnit=on
  Calc_RMSE_BROS2 : MATLAB Function  TreatAsAtomicUnit=on
  RMSE_BROS1 : Outport
  RMSE_BROS2 : Outport  Port=2
  wires:
  error_BROS1/1 -> Calc_RMSE_BROS1/1(error)
  Calc_RMSE_BROS1/1(RMSE) -> RMSE_BROS1/1
  Calc_RMSE_BROS2/1(RMSE) -> RMSE_BROS2/1
  error_BROS2/1 -> Calc_RMSE_BROS2/1(error)

== system model_base_bros/Experiment & Haptics/Trial Logic ==
  Trial Start Signal : Inport
  Trial Done Signal : Inport  Port=2
  CheckTrialIsRunning : simulink_extras/Flip Flops/S-R Flip-Flop  initial_condition=0
  Data Type Conversion : DataTypeConversion  OutDataTypeStr=double
  Detect Rise Positive : simulink/Logic and Bit Operations/Detect Rise Positive  vinit=0  OutDataTypeStr=boolean
  Detect Rise Positive1 : simulink/Logic and Bit Operations/Detect Rise Positive  vinit=0  OutDataTypeStr=boolean
  Logical Operator : Logic  AllPortsSameDT=off  OutDataTypeStr=boolean
  Memory : Memory
  StopWatch : Subsystem
  Terminator4 : Terminator
  TrialTime : Outport
  TrialRunning : Outport  Port=2
  wires:
  CheckTrialIsRunning/1 -> Memory/1, Data Type Conversion/1
  Memory/1 -> StopWatch/Enable, Logical Operator/1
  Trial Start Signal/1 -> Detect Rise Positive/1
  Detect Rise Positive1/1 -> CheckTrialIsRunning/2
  Detect Rise Positive/1 -> CheckTrialIsRunning/1
  StopWatch/1(trialTime) -> TrialTime/1
  CheckTrialIsRunning/2 -> Terminator4/1
  Data Type Conversion/1 -> TrialRunning/1
  Trial Done Signal/1 -> Logical Operator/2
  Logical Operator/1 -> Detect Rise Positive1/1

== system model_base_bros/Robot1/AppendToLoggerBus ==
  BusRobot : Inport
  ToEtherCAT_ToLogger : Inport  Port=2
  Controller_ToLogger : Inport  Port=3
  SystemState : Inport  Port=4
  Bus Creator : BusCreator  Inputs=8
  Bus Selector : BusSelector  OutputSignals=xOpSpace,qJointSpace,BusFTSensor,BusActuators
  Bus Selector1 : BusSelector  OutputSignals=ToEtherCAT_ToLogger_Actuator1,ToEtherCAT_ToLogger_Actuator2
  ToLogger : Outport
  wires:
  Bus Creator/1 -> ToLogger/1  "LoggerBus"
  Bus Selector/4 -> Bus Creator/4  "<BusActuators>"
  Bus Selector/1 -> Bus Creator/1  "<xOpSpace>"
  Bus Selector/3 -> Bus Creator/3  "<BusFTSensor>"
  Bus Selector/2 -> Bus Creator/2  "<qJointSpace>"
  BusRobot/1 -> Bus Selector/1
  ToEtherCAT_ToLogger/1 -> Bus Selector1/1
  Bus Selector1/1 -> Bus Creator/5  "<ToEtherCAT_ToLogger_Actuator1>"
  Bus Selector1/2 -> Bus Creator/6  "<ToEtherCAT_ToLogger_Actuator2>"
  Controller_ToLogger/1 -> Bus Creator/7
  SystemState/1 -> Bus Creator/8  "SystemState"

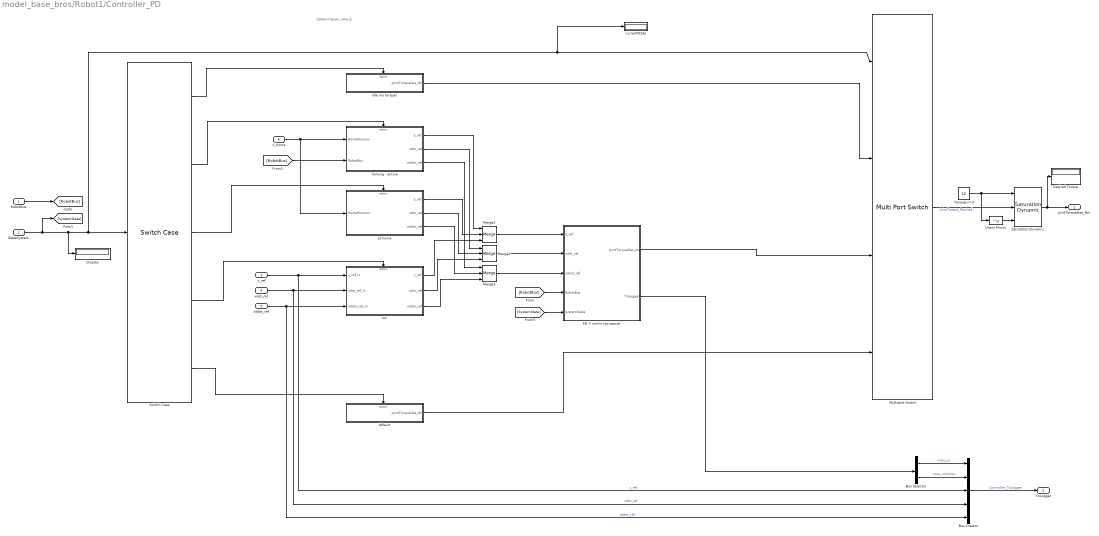
== system model_base_bros/Robot1/Controller_PD ==
  note: OPERATIONAL SPACE
  RobotBus : Inport
  StateSystem : Inport  Port=2
  x_ref : Inport  Port=3
  xdot_ref : Inport  Port=4
  xddot_ref : Inport  Port=5
  x_home : Inport  Port=6
  Bus Creator : BusCreator  Inputs=5
  Bus Selector : BusSelector  OutputSignals=tau_y,tau_nlcomp
  Desired Torque : Display
  Display : Display
  Merge1 : Merge  Inputs=3  InitialOutput=[0;0]
  Merge2 : Merge  Inputs=3  InitialOutput=[0;0]
  Merge3 : Merge  Inputs=3  InitialOutput=[0;0]
  Multiport Switch : MultiPortSwitch  DataPortOrder=Specify indices  Inputs=4  DataPortIndices={[0,1,2,201,299,301],[302,399,4]}  DataPortForDefault=Additional data port
  PD + nonlin (op space) : Subsystem
  Saturation Dynamic : simulink/Discontinuities/Saturation Dynamic  OutMin=[]  OutMax=[]  OutDataTypeStr=Inherit: Same as second input  OutDataType=fixdt(1, 16)  OutScaling=2^-10  DoSatur=off
  Switch Case : SwitchCase  CaseConditions={[0,1,2,201,299,301],302, 399,[4]}
  TorqueLimit : Constant  Value=12
  Unary Minus : UnaryMinus
  at home : Subsystem
  currentState : Display
  default : Subsystem  TreatAsAtomicUnit=on
  homing - active : Subsystem
  idle (no torque) : Subsystem  TreatAsAtomicUnit=on
  run : Subsystem
  JointTorqueDes_Nm : Outport
  ToLogger : Outport  Port=2
  wires:
  [SystemState] -> PD + nonlin (op space)/5(systemState)
  xddot_ref/1 -> Bus Creator/5, run/3(xddot_ref_in)  "xddot_ref"
  xdot_ref/1 -> Bus Creator/4, run/2(xdot_ref_in)  "xdot_ref"
  x_ref/1 -> Bus Creator/3, run/1(x_ref_in)  "x_ref"
  [RobotBus] -> PD + nonlin (op space)/4(RobotBus)
  RobotBus/1 -> [RobotBus]
  Merge3/1 -> PD + nonlin (op space)/3(xddot_ref)
  Merge2/1 -> PD + nonlin (op space)/2(xdot_ref)
  Merge1/1 -> PD + nonlin (op space)/1(x_ref)
  idle (no torque)/1(JointTorqueDes_Nm) -> Multiport Switch/2
  Switch Case/2 -> homing - active/Action
  Switch Case/1 -> idle (no torque)/Action
  default/1(JointTorqueDes_Nm) -> Multiport Switch/4
  Switch Case/5 -> default/Action
  Saturation Dynamic/1 -> Desired Torque/1, JointTorqueDes_Nm/1
  Switch Case/3 -> at home/Action
  homing - active/1(x_ref) -> Merge1/1
  run/1(x_ref) -> Merge1/3
  StateSystem/1 -> Display/1, Multiport Switch/1, currentState/1, Switch Case/1, [SystemState]
  run/2(xdot_ref) -> Merge2/3
  run/3(xddot_ref) -> Merge3/3
  homing - active/2(xdot_ref) -> Merge2/1
  homing - active/3(xddot_ref) -> Merge3/1
  Multiport Switch/1 -> Saturation Dynamic/2  "JointTorque_Desired"
  PD + nonlin (op space)/2(ToLogger) -> Bus Selector/1
  x_home/1 -> at home/1(HomePosition), homing - active/1(HomePosition)
  Bus Creator/1 -> ToLogger/1  "Controller_ToLogger"
  Bus Selector/1 -> Bus Creator/1  "<tau_y>"
  Bus Selector/2 -> Bus Creator/2  "<tau_nlcomp>"
  TorqueLimit/1 -> Unary Minus/1, Saturation Dynamic/1
  Unary Minus/1 -> Saturation Dynamic/3
  [RobotBus] -> homing - active/2(RobotBus)
  at home/1(x_ref) -> Merge1/2
  at home/2(xdot_ref) -> Merge2/2
  at home/3(xddot_ref) -> Merge3/2
  Switch Case/4 -> run/Action
  PD + nonlin (op space)/1(JointTorqueDes_Nm) -> Multiport Switch/3

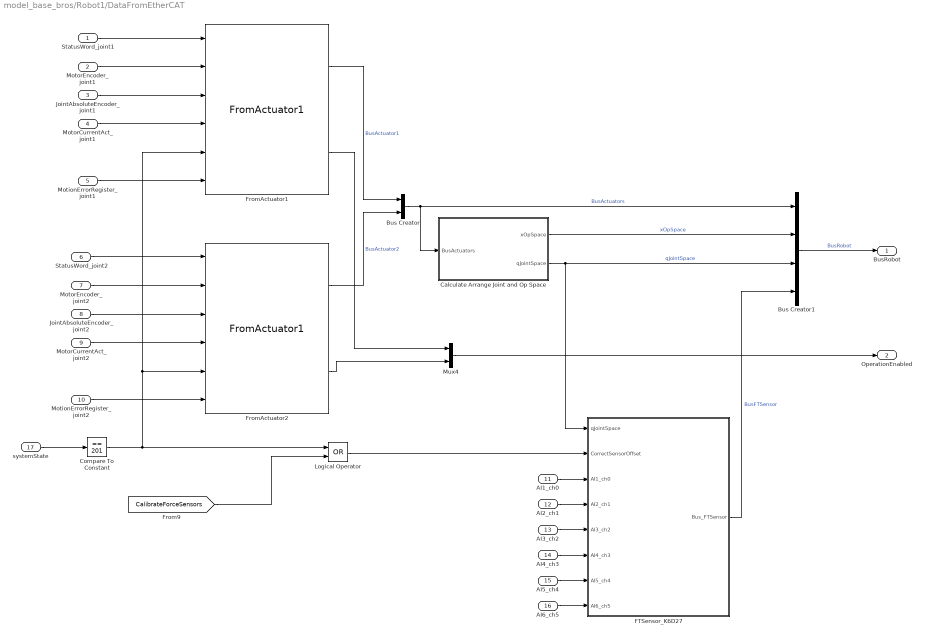
== system model_base_bros/Robot1/DataFromEtherCAT ==
  StatusWord_joint1 : Inport
  MotorEncoder_joint1 : Inport  Port=2
  JointAbsoluteEncoder_joint1 : Inport  Port=3
  MotorCurrentAct_joint1 : Inport  Port=4
  MotionErrorRegister_joint1 : Inport  Port=5  OutDataTypeStr=uint16
  StatusWord_joint2 : Inport  Port=6
  MotorEncoder_joint2 : Inport  Port=7
  "JointAbsoluteEncoder_joint2 " : Inport  Port=8
  MotorCurrentAct_joint2 : Inport  Port=9
  MotionErrorRegister_joint2 : Inport  Port=10  OutDataTypeStr=uint16
  AI1_ch0 : Inport  Port=11
  AI2_ch1 : Inport  Port=12
  AI3_ch2 : Inport  Port=13
  AI4_ch3 : Inport  Port=14
  AI5_ch4 : Inport  Port=15
  AI6_ch5 : Inport  Port=16
  systemState : Inport  Port=17
  Bus Creator : BusCreator  Inputs=2
  Bus Creator1 : BusCreator  Inputs=4
  Calculate Arrange Joint and Op Space : Subsystem
  Compare To Constant : simulink/Logic and Bit Operations/Compare To Constant  relop===  const=201  OutDataTypeStr=boolean
  FTSensor_K6D27 : Subsystem  mask{FTSensorStruct=RobotStruct.FTSensor}
      mask prompts: FTSensorStruct "Struct for force torque sensor"
  FromActuator1 : LibraryFM/FromActuator1  ActuatorStruct=RobotStruct.Actuator1
  FromActuator2 : LibraryFM/FromActuator1  ActuatorStruct=RobotStruct.Actuator2
  Logical Operator : Logic  Operator=OR  AllPortsSameDT=off  OutDataTypeStr=boolean
  Mux4 : Mux  Inputs=2
  BusRobot : Outport
  OperationEnabled : Outport  Port=2
  wires:
  FTSensor_K6D27/1(Bus_FTSensor) -> Bus Creator1/4  "BusFTSensor"
  FromActuator1/1 -> Bus Creator/1  "BusActuator1"
  FromActuator2/1 -> Bus Creator/2  "BusActuator2"
  FromActuator1/2 -> Mux4/1
  Mux4/1 -> OperationEnabled/1
  FromActuator2/2 -> Mux4/2
  MotorEncoder_joint1/1 -> FromActuator1/2
  StatusWord_joint1/1 -> FromActuator1/1
  JointAbsoluteEncoder_joint1/1 -> FromActuator1/3
  MotorCurrentAct_joint1/1 -> FromActuator1/4
  MotorEncoder_joint2/1 -> FromActuator2/2
  StatusWord_joint2/1 -> FromActuator2/1
  "JointAbsoluteEncoder_joint2 "/1 -> FromActuator2/3
  MotorCurrentAct_joint2/1 -> FromActuator2/4
  Bus Creator/1 -> Calculate Arrange Joint and Op Space/1(BusActuators), Bus Creator1/1  "BusActuators"
  Bus Creator1/1 -> BusRobot/1  "BusRobot"
  Calculate Arrange Joint and Op Space/2(qJointSpace) -> FTSensor_K6D27/1(qJointSpace), Bus Creator1/3  "qJointSpace"
  systemState/1 -> Compare To Constant/1
  AI1_ch0/1 -> FTSensor_K6D27/3(AI1_ch0)
  AI2_ch1/1 -> FTSensor_K6D27/4(AI2_ch1)
  AI3_ch2/1 -> FTSensor_K6D27/5(AI3_ch2)
  AI4_ch3/1 -> FTSensor_K6D27/6(AI4_ch3)
  AI5_ch4/1 -> FTSensor_K6D27/7(AI5_ch4)
  AI6_ch5/1 -> FTSensor_K6D27/8(AI6_ch5)
  Compare To Constant/1 -> Logical Operator/1, FromActuator1/5, FromActuator2/5
  Calculate Arrange Joint and Op Space/1(xOpSpace) -> Bus Creator1/2  "xOpSpace"
  [CalibrateForceSensors] -> Logical Operator/2
  Logical Operator/1 -> FTSensor_K6D27/2(CorrectSensorOffset)
  MotionErrorRegister_joint1/1 -> FromActuator1/6
  MotionErrorRegister_joint2/1 -> FromActuator2/6

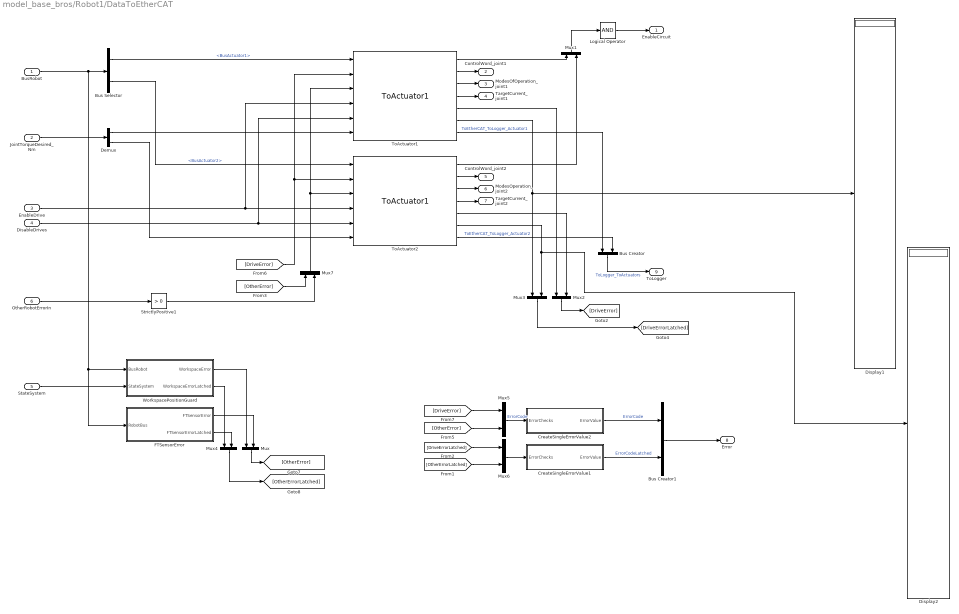
== system model_base_bros/Robot1/DataToEtherCAT ==
  BusRobot : Inport
  JointTorqueDesired_Nm : Inport  Port=2
  EnableDrive : Inport  Port=3
  DisableDrives : Inport  Port=4
  StateSystem : Inport  Port=5
  OtherRobotErrorIn : Inport  Port=6
  Bus Creator : BusCreator  Inputs=2
  Bus Creator1 : BusCreator  Inputs=2
  Bus Selector : BusSelector  OutputSignals=BusActuators.BusActuator1,BusActuators.BusActuator2
  CreateSingleErrorValue1 : Subsystem
  CreateSingleErrorValue2 : Subsystem
  Demux : Demux  Outputs=2
  Display1 : Display
  Display2 : Display
  FTSensorError : Subsystem
  Logical Operator : Logic  Inputs=1  AllPortsSameDT=off  OutDataTypeStr=boolean
  Mux{,1..7} (8 alike) : Mux  Inputs=2
  StrictlyPositive1 : simulink/Logic and Bit Operations/Compare To Zero  relop=>  OutDataTypeStr=boolean
  ToActuator1 : LibraryFM/ToActuator1  ActuatorStruct=RobotStruct.Actuator1
  ToActuator2 : LibraryFM/ToActuator1  ActuatorStruct=RobotStruct.Actuator2
  WorkspacePositionGuard : Subsystem
  EnableCircuit : Outport  OutDataTypeStr=boolean
  ControlWord_joint1 : Outport  Port=2  OutDataTypeStr=uint16
  ModesOfOperation_joint1 : Outport  Port=3  OutDataTypeStr=int8
  TargetCurrent_joint1 : Outport  Port=4  OutDataTypeStr=int16
  ControlWord_joint2 : Outport  Port=5  OutDataTypeStr=uint16
  ModesOperation_joint2 : Outport  Port=6  OutDataTypeStr=int8
  TargetCurrent_joint2 : Outport  Port=7  OutDataTypeStr=int16
  Error : Outport  Port=8
  ToLogger : Outport  Port=9
  wires:
  Bus Creator/1 -> ToLogger/1  "ToLogger_ToActuators"
  ToActuator2/7 -> Bus Creator/2  "ToEtherCAT_ToLogger_Actuator2"
  ToActuator1/7 -> Bus Creator/1  "ToEtherCAT_ToLogger_Actuator1"
  ToActuator1/5 -> Mux2/1
  ToActuator2/5 -> Mux2/2
  Mux2/1 -> [DriveError]
  ToActuator1/6 -> Display1/1, Mux3/1
  ToActuator2/6 -> Display2/1, Mux3/2
  [DriveError] -> ToActuator1/2, ToActuator2/2
  Mux1/1 -> Logical Operator/1
  ToActuator1/1 -> Mux1/1
  ToActuator2/1 -> Mux1/2
  ToActuator1/2 -> ControlWord_joint1/1
  ToActuator1/3 -> ModesOfOperation_joint1/1
  ToActuator2/2 -> ControlWord_joint2/1
  ToActuator1/4 -> TargetCurrent_joint1/1
  ToActuator2/4 -> TargetCurrent_joint2/1
  ToActuator2/3 -> ModesOperation_joint2/1
  Logical Operator/1 -> EnableCircuit/1
  Demux/2 -> ToActuator2/6
  JointTorqueDesired_Nm/1 -> Demux/1
  Demux/1 -> ToActuator1/6
  BusRobot/1 -> WorkspacePositionGuard/1(BusRobot), FTSensorError/1(RobotBus), Bus Selector/1
  Bus Selector/2 -> ToActuator2/1  "<BusActuator2>"
  Bus Selector/1 -> ToActuator1/1  "<BusActuator1>"
  DisableDrives/1 -> ToActuator1/5, ToActuator2/5
  EnableDrive/1 -> ToActuator1/4, ToActuator2/4
  Mux3/1 -> [DriveErrorLatched]
  StateSystem/1 -> WorkspacePositionGuard/2(StateSystem)
  FTSensorError/1(FTSensorError) -> Mux/2
  FTSensorError/2(FTSensorErrorLatched) -> Mux4/2
  WorkspacePositionGuard/1(WorkspaceError) -> Mux/1
  WorkspacePositionGuard/2(WorkspaceErrorLatched) -> Mux4/1
  Mux/1 -> [OtherError]
  Mux4/1 -> [OtherErrorLatched]
  [DriveError] -> Mux5/1
  [OtherError] -> Mux5/2
  CreateSingleErrorValue1/1(ErrorValue) -> Bus Creator1/2  "ErrorCodeLatched"
  [DriveErrorLatched] -> Mux6/1
  [OtherErrorLatched] -> Mux6/2
  Mux6/1 -> CreateSingleErrorValue1/1(ErrorChecks)
  Mux5/1 -> CreateSingleErrorValue2/1(ErrorChecks)  "ErrorCode"
  Bus Creator1/1 -> Error/1
  CreateSingleErrorValue2/1(ErrorValue) -> Bus Creator1/1  "ErrorCode"
  [OtherError] -> Mux7/1
  Mux7/1 -> ToActuator2/3, ToActuator1/3
  OtherRobotErrorIn/1 -> StrictlyPositive1/1
  StrictlyPositive1/1 -> Mux7/2

== system model_base_bros/Robot2/AppendToLoggerBus ==
  BusRobot : Inport
  ToEtherCAT_ToLogger : Inport  Port=2
  Controller_ToLogger : Inport  Port=3
  SystemState : Inport  Port=4
  Bus Creator : BusCreator  Inputs=8
  Bus Selector : BusSelector  OutputSignals=xOpSpace,qJointSpace,BusFTSensor,BusActuators
  Bus Selector1 : BusSelector  OutputSignals=ToEtherCAT_ToLogger_Actuator1,ToEtherCAT_ToLogger_Actuator2
  ToLogger : Outport
  wires:
  Bus Creator/1 -> ToLogger/1  "LoggerBus"
  Bus Selector/4 -> Bus Creator/4  "<BusActuators>"
  Bus Selector/1 -> Bus Creator/1  "<xOpSpace>"
  Bus Selector/3 -> Bus Creator/3  "<BusFTSensor>"
  Bus Selector/2 -> Bus Creator/2  "<qJointSpace>"
  BusRobot/1 -> Bus Selector/1
  ToEtherCAT_ToLogger/1 -> Bus Selector1/1
  Bus Selector1/1 -> Bus Creator/5  "<ToEtherCAT_ToLogger_Actuator1>"
  Bus Selector1/2 -> Bus Creator/6  "<ToEtherCAT_ToLogger_Actuator2>"
  Controller_ToLogger/1 -> Bus Creator/7
  SystemState/1 -> Bus Creator/8  "SystemState"
